simulink model "sim"  (R2022a)
settings: Solver=VariableStepAuto  StartTime=0.0  StopTime=3  RelTol=1e-3
values from neighbouring files (symbols this model uses):
  C1 = minreal ((1/Gzas)* (Gcl/(1-Gcl)))    [ES2.m]
  C2 = minreal ((1/Gzas)* (Gcl/(1-Gcl)))    [ES2.m]
  Gzas = tf(num, den,Tc)    [ES2.m]
  Tc = 0.1    [ES2.m]
settings Model: Creator=Stefano  LastModifiedBy=Stefano

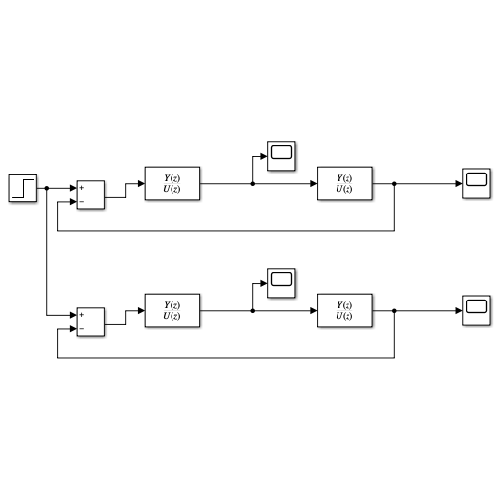
[thumbnail: Simulink's stored preview of the top-level diagram]
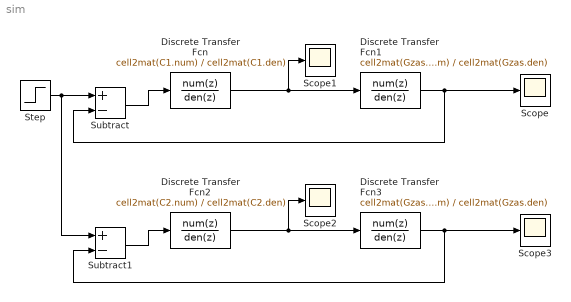
== system sim ==
  Discrete Transfer Fcn : DiscreteTransferFcn  Numerator=cell2mat(C1.num)  Denominator=cell2mat(C1.den)  SampleTime=Tc
  Discrete Transfer Fcn1 : DiscreteTransferFcn  Numerator=cell2mat(Gzas.num)  Denominator=cell2mat(Gzas.den)  SampleTime=Tc
  Discrete Transfer Fcn2 : DiscreteTransferFcn  Numerator=cell2mat(C2.num)  Denominator=cell2mat(C2.den)  SampleTime=Tc
  Discrete Transfer Fcn3 : DiscreteTransferFcn  Numerator=cell2mat(Gzas.num)  Denominator=cell2mat(Gzas.den)  SampleTime=Tc
  Scope{,1..3} (4 alike) : Scope
  Step : Step  SampleTime=0
  Subtract : Sum  Inputs=+-
  Subtract1 : Sum  Inputs=+-
  wires:
  Step/1 -> Subtract1/1, Subtract/1
  Subtract/1 -> Discrete Transfer Fcn/1
  Discrete Transfer Fcn/1 -> Scope1/1, Discrete Transfer Fcn1/1
  Discrete Transfer Fcn1/1 -> Subtract/2, Scope/1
  Discrete Transfer Fcn2/1 -> Scope2/1, Discrete Transfer Fcn3/1
  Subtract1/1 -> Discrete Transfer Fcn2/1
  Discrete Transfer Fcn3/1 -> Scope3/1, Subtract1/2
